simulink model "PID_Roll"  (R2016b)
settings: Solver=ode3  StartTime=0.0  StopTime=20  FixedStep=.02  RelTol=1e-3  EnableMultiTasking=on
InitFcn:
  | close all
  | clear
  | clc
  | Parameter_Modeling
  | ST=0.02;
  | angle_scale=.0109863;  % 1/91.0222
  | time_scale=.01;
undefined symbols (not defined in the file or in its folder): KD_Roll, KI_Roll, KP_Roll
libraries: arduinolib x5
settings Model: SimulationMode=external  ExtModeTrigDuration=2  Creator=Alireza  LastModifiedBy=Ali
settings DataIOCC: LimitDataPoints=on  SaveFormat=Array
settings OptimizationCC: ExpressionDepthLimit=2147483647  MaxStackSize=64
settings DebuggingCC: UnderspecifiedInitializationDetection=Classic  MergeDetectMultiDrivingBlocksExec=none  ParameterTunabilityLossMsg=error  StateNameClashWarn=warning  SFUnexpectedBacktrackingDiag=warning  SFNoUnconditionalDefaultTransitionDiag=warning  SFExecutionAtInitializationDiag=none
settings HardwareCC: ProdBitPerInt=16  ProdBitPerPointer=16  ProdBitPerSizeT=16  ProdBitPerPtrDiffT=16  ProdLargestAtomicFloat=None  ProdWordSize=8  ProdHWDeviceType=Atmel->AVR
settings ModelReferenceCC: PropagateSignalLabelsOutOfModel=off
settings RTWCC: Description=Embedded Coder  SystemTargetFile=ert.tlc  HardwareBoard=Arduino Mega 2560  TLCOptions=-aInlineSetEventsForThisBaseRateFcn=TLC_FALSE -aRateBasedStepFcn=1 -aSuppressMultiTaskScheduler=TLC_FALSE  TemplateMakefile=ert_default_tmf  GenerateReport=on  RTWVerbose=off  Toolchain=Arduino AVR  BuildConfiguration=Faster Runs  IncludeHyperlinkInReport=on  LaunchReport=on  GenerateTraceInfo=on  GenerateTraceReport=on  GenerateTraceReportSl=on  GenerateTraceReportSf=on  GenerateTraceReportEml=on
settings CodeAppCC: ForceParamTrailComments=on  IgnoreCustomStorageClasses=off  OperatorAnnotations=on  SimulinkDataObjDesc=on  SFDataObjDesc=on  MATLABFcnDesc=on  CustomSymbolStrType=$N$R$M  InsertBlockDesc=on  MATLABSourceComments=on  InternalIdentifier=Classic
settings ERTTargetCC: SupportContinuousTime=on  SupportVariableSizeSignals=on
settings ConfigComp: CovMetricSettings=dw  CovHtmlReporting=on  CovSaveCumulativeToWorkspaceVar=on  CovSaveSingleToWorkspaceVar=on  CovExternalEMLEnable=off  CovSFcnEnable=off

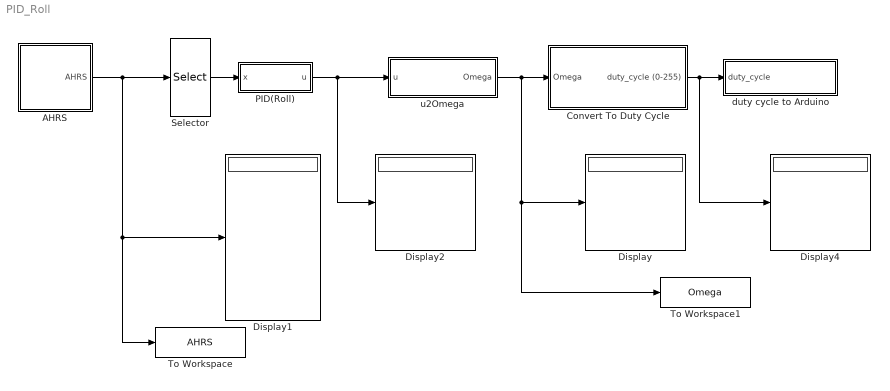
== system PID_Roll ==
  AHRS : Subsystem
      mask Display: image('UM7.jpg'); % Use "Edit Image" on toolstrip to change.
  Convert To Duty Cycle : Subsystem
  Display{,1..2,4} (4 alike) : Display
  PID(Roll) : Subsystem
  Selector : Selector  InputPortWidth=6  IndexOptions=Index vector (dialog)  Indices=[1 4]  OutputSizes=1
  To Workspace : ToWorkspace  VariableName=AHRS  SaveFormat=Timeseries  SampleTime=-1
  To Workspace1 : ToWorkspace  VariableName=Omega  SaveFormat=Timeseries  SampleTime=-1
  duty cycle to Arduino : Subsystem
  u2Omega : Subsystem
  wires:
  u2Omega/1(Omega) -> To Workspace1/1, Display/1, Convert To Duty Cycle/1(Omega)
  PID(Roll)/1(u) -> Display2/1, u2Omega/1(u)
  AHRS/1(AHRS) -> Selector/1, To Workspace/1, Display1/1
  Convert To Duty Cycle/1(duty_cycle (0-255)) -> Display4/1, duty cycle to Arduino/1(duty_cycle)
  Selector/1 -> PID(Roll)/1(x)

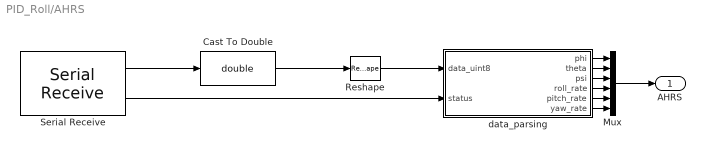
== system PID_Roll/AHRS ==
  Cast To Double : DataTypeConversion  OutDataTypeStr=double
  Mux : Mux  Inputs=6
  Reshape : Reshape
  Serial Receive : arduinolib/Serial Receive  isARMArch=off  portNumber=1  DataType=uint8  Datalength=32  SampleTime=0.02  showOutStatus=on  blockPlatform=arduino
  data_parsing : MATLAB Function  TreatAsAtomicUnit=on
  AHRS : Outport
  wires:
  data_parsing/2(theta) -> Mux/2
  data_parsing/3(psi) -> Mux/3
  data_parsing/4(roll_rate) -> Mux/4
  Reshape/1 -> data_parsing/1(data_uint8)
  data_parsing/5(pitch_rate) -> Mux/5
  Serial Receive/2 -> data_parsing/2(status)
  data_parsing/6(yaw_rate) -> Mux/6
  Cast To Double/1 -> Reshape/1
  Serial Receive/1 -> Cast To Double/1
  data_parsing/1(phi) -> Mux/1
  Mux/1 -> AHRS/1

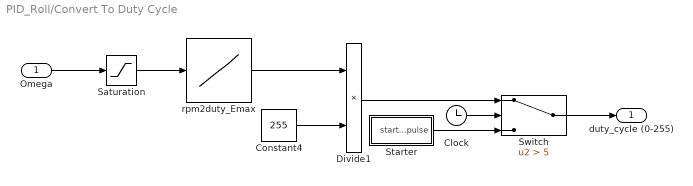
== system PID_Roll/Convert To Duty Cycle ==
  Omega : Inport
  Clock : Clock
  Constant4 : Constant  Value=255
  Divide1 : Product  Inputs=**
  Saturation : Saturate  UpperLimit=6000  LowerLimit=1300
  Starter : Subsystem
  Switch : Switch  Criteria=u2 > Threshold  Threshold=5
  rpm2duty_Emax : Lookup_n-D  NumberOfTableDimensions=1  BreakpointsForDimension1=|  Table=|  RndMeth=Simplest  InputSameDT=on
      BreakpointsForDimension1=|
      | [1201
      | 2305
      | 3096
      | 3930
      | 4118
      | 4555
      | 5122
      | 5552
      | 5957
      | 6291
      | 6360]
      Table=|
      | [0.5
      | 0.55
      | 0.6
      | 0.65
      | 0.7
      | 0.75
      | 0.8
      | 0.85
      | 0.9
      | 0.95
      | 1]
  duty_cycle (0-255) : Outport
  wires:
  Switch/1 -> duty_cycle (0-255)/1
  Clock/1 -> Switch/2
  Divide1/1 -> Switch/1
  rpm2duty_Emax/1 -> Divide1/1
  Starter/1(start_pulse) -> Switch/3
  Omega/1 -> Saturation/1
  Constant4/1 -> Divide1/2
  Saturation/1 -> rpm2duty_Emax/1

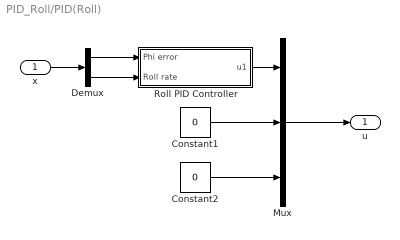
== system PID_Roll/PID(Roll) ==
  x : Inport
  Constant1 : Constant  Value=0
  Constant2 : Constant  Value=0
  Demux : Demux  Outputs=2
  Mux : Mux  Inputs=3
  Roll PID Controller : Subsystem  VariantControl=Choice
  u : Outport
  wires:
  Mux/1 -> u/1
  x/1 -> Demux/1
  Demux/2 -> Roll PID Controller/2(Roll rate)
  Constant2/1 -> Mux/3
  Demux/1 -> Roll PID Controller/1(Phi error)
  Roll PID Controller/1(u1) -> Mux/1
  Constant1/1 -> Mux/2

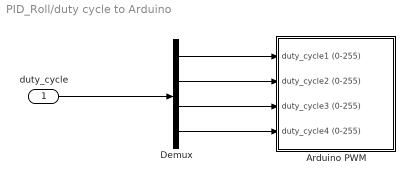
== system PID_Roll/duty cycle to Arduino ==
  duty_cycle : Inport
  Arduino PWM : Subsystem  mask{Motor1=8, Motor2=9, Motor3=10, Motor4=11}
      mask prompts: Motor1 "Motor 1 Pin Number"; Motor2 "Motor 2 Pin Number"; Motor3 "Motor 3 Pin Number"; Motor4 "Motor 4 Pin Number"
  Demux : Demux
  wires:
  duty_cycle/1 -> Demux/1
  Demux/1 -> Arduino PWM/1(duty_cycle1 (0-255))
  Demux/2 -> Arduino PWM/2(duty_cycle2 (0-255))
  Demux/3 -> Arduino PWM/3(duty_cycle3 (0-255))
  Demux/4 -> Arduino PWM/4(duty_cycle4 (0-255))

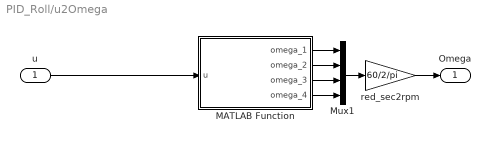
== system PID_Roll/u2Omega ==
  u : Inport
  MATLAB Function : MATLAB Function  TreatAsAtomicUnit=on
  Mux1 : Mux
  red_sec2rpm : Gain  Gain=60/2/pi
  Omega : Outport
  wires:
  Mux1/1 -> red_sec2rpm/1
  MATLAB Function/2(omega_2) -> Mux1/2
  u/1 -> MATLAB Function/1(u)
  MATLAB Function/3(omega_3) -> Mux1/3
  MATLAB Function/1(omega_1) -> Mux1/1
  MATLAB Function/4(omega_4) -> Mux1/4
  red_sec2rpm/1 -> Omega/1

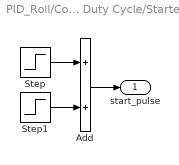
== system PID_Roll/Convert To Duty Cycle/Starter ==
  Add : Sum
  Step : Step  After=140
  Step1 : Step  Time=2  After=-30
  start_pulse : Outport
  wires:
  Add/1 -> start_pulse/1
  Step/1 -> Add/1
  Step1/1 -> Add/2

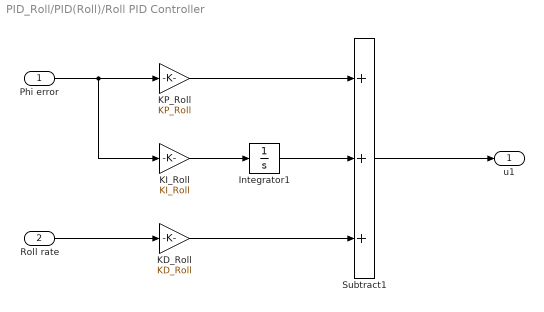
== system PID_Roll/PID(Roll)/Roll PID Controller ==
  Phi error : Inport
  Roll rate : Inport  Port=2
  Integrator1 : Integrator
  KD_Roll : Gain  Gain=KD_Roll
  KI_Roll : Gain  Gain=KI_Roll
  KP_Roll : Gain  Gain=KP_Roll
  Subtract1 : Sum  Inputs=+++
  u1 : Outport
  wires:
  Integrator1/1 -> Subtract1/2
  KI_Roll/1 -> Integrator1/1
  KD_Roll/1 -> Subtract1/3
  Subtract1/1 -> u1/1
  KP_Roll/1 -> Subtract1/1
  Roll rate/1 -> KD_Roll/1
  Phi error/1 -> KI_Roll/1, KP_Roll/1

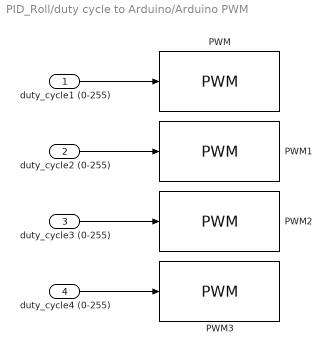
== system PID_Roll/duty cycle to Arduino/Arduino PWM ==
  duty_cycle1 (0-255) : Inport
  duty_cycle2 (0-255) : Inport  Port=2
  duty_cycle3 (0-255) : Inport  Port=3
  duty_cycle4 (0-255) : Inport  Port=4
  PWM : arduinolib/PWM  pinNumber=Motor1  frequencyType=Default  desiredFrequency=490.2  achievableFrequency=490.2
  PWM1 : arduinolib/PWM  pinNumber=Motor2  frequencyType=Default  desiredFrequency=490.2  achievableFrequency=490.2
  PWM2 : arduinolib/PWM  pinNumber=Motor3  frequencyType=Default  desiredFrequency=490.2  achievableFrequency=490.2
  PWM3 : arduinolib/PWM  pinNumber=Motor4  frequencyType=Default  desiredFrequency=490.2  achievableFrequency=490.2
  wires:
  duty_cycle1 (0-255)/1 -> PWM/1
  duty_cycle2 (0-255)/1 -> PWM1/1
  duty_cycle3 (0-255)/1 -> PWM2/1
  duty_cycle4 (0-255)/1 -> PWM3/1

== matlab function PID_Roll/AHRS/data_parsing ==
  data: phi output size=1; data_uint8 input size=32; theta output size=1; psi output size=1; roll_rate output size=1; pitch_rate output size=1; yaw_rate output size=1; status input
function [phi,theta,psi,roll_rate,pitch_rate,yaw_rate] = fcn(data_uint8, status)
persistent stepp check_sum...
    phi_p theta_p psi_p roll_rate_p pitch_rate_p yaw_rate_p...
    phi_last theta_last psi_last roll_rate_last pitch_rate_last yaw_rate_last;
%% Initialize
if isempty(stepp)
    stepp=0;
    check_sum=0;
    phi_p=0;
    theta_p=0;
    psi_p=0;
    roll_rate_p=0;
    pitch_rate_p=0;
    yaw_rate_p=0;
    phi_last=0;
    theta_last=0;
    psi_last=0;
    roll_rate_last=0;
    pitch_rate_last=0;
    yaw_rate_last=0;
end
angle_scale=.0109863;  % 1/91.0222
rate_scale=1/16;
%% Check Each Byte
if status
    for i = 1:length(data_uint8)
        if (data_uint8(i)==115 && stepp==0)
            stepp=1;
            check_sum=data_uint8(i);
        elseif(stepp==1 && data_uint8(i)==110)
            stepp=stepp+1;
            check_sum=check_sum+data_uint8(i);
        elseif(stepp==2 && data_uint8(i)==112)
            stepp=stepp+1;
            check_sum=check_sum+data_uint8(i);
        elseif(stepp==3 && data_uint8(i)==212)
            stepp=stepp+1;
            check_sum=check_sum+data_uint8(i);
        elseif(stepp==4 && data_uint8(i)==112)
            stepp=stepp+1;
            check_sum=check_sum+data_uint8(i);
        elseif(stepp==5)
            phi_p=data_uint8(i)*256;
            stepp=stepp+1;
            check_sum=check_sum+data_uint8(i);
        elseif(stepp==6)
            phi_p=phi_p+data_uint8(i);
            stepp=stepp+1;
            check_sum=check_sum+data_uint8(i);
        elseif(stepp==7)
            theta_p=data_uint8(i)*256;
            stepp=stepp+1;
            check_sum=check_sum+data_uint8(i);
        elseif(stepp==8)
            theta_p=theta_p+data_uint8(i);
            stepp=stepp+1;
            check_sum=check_sum+data_uint8(i);
        elseif(stepp==9)
            psi_p=data_uint8(i)*256;
            stepp=stepp+1;
            check_sum=check_sum+data_uint8(i);
        elseif(stepp==10)
            psi_p=psi_p+data_uint8(i);
            stepp=stepp+1;
            check_sum=check_sum+data_uint8(i);
        elseif(stepp==11 || stepp==12)
            if(data_uint8(i)==0)
                stepp=stepp+1;
            else
                stepp=0;
            end
        elseif(stepp==13)
            roll_rate_p=data_uint8(i)*256;
            stepp=stepp+1;
            check_sum=check_sum+data_uint8(i);
        elseif(stepp==14)
            roll_rate_p=roll_rate_p+data_uint8(i);
            stepp=stepp+1;
            check_sum=check_sum+data_uint8(i);
        elseif(stepp==15)
            pitch_rate_p=data_uint8(i)*256;
            stepp=stepp+1;
            check_sum=check_sum+data_uint8(i);
        elseif(stepp==16)
            pitch_rate_p=pitch_rate_p+data_uint8(i);
            stepp=stepp+1;
            check_sum=check_sum+data_uint8(i);
        elseif(stepp==17)
            yaw_rate_p=data_uint8(i)*256;
            stepp=stepp+1;
            check_sum=check_sum+data_uint8(i);
        elseif(stepp==18)
            yaw_rate_p=yaw_rate_p+data_uint8(i);
            stepp=stepp+1;
            check_sum=check_sum+data_uint8(i);
        elseif(stepp==19 || stepp==20)
            if(data_uint8(i)==0)
                stepp=stepp+1;
            else
                stepp=0;
            end
        elseif(stepp==21 || stepp==22 || stepp==23 || stepp==24)
            stepp=stepp+1;
            check_sum=check_sum+data_uint8(i);
        elseif(stepp==25)
            if (floor(check_sum/256)==data_uint8(i))
                stepp=stepp+1;
            else
                stepp=0;
            end
        elseif(stepp==26)
            if(mod(check_sum,256)==data_uint8(i))
                phi_last=double(typecast(uint16(phi_p), 'int16'))*angle_scale;
                if mod(phi_last,360)>180
                    phi_last=mod(phi_last,360)-360;
                else
                    phi_last=mod(phi_last,360);
                end
                theta_last=double(typecast(uint16(theta_p), 'int16'))*angle_scale;
                if mod(theta_last,360)>180
                    theta_last=mod(theta_last,360)-360;
                else
                    theta_last=mod(theta_last,360);
                end
                psi_last=double(typecast(uint16(psi_p), 'int16'))*angle_scale;
                if mod(psi_last,360)>180
                    psi_last=mod(psi_last,360)-360;
                else
                    psi_last=mod(psi_last,360);
                end
                roll_rate_last=double(typecast(uint16(roll_rate_p), 'int16'))*rate_scale;
                if mod(roll_rate_last,360)>180
                    roll_rate_last=mod(roll_rate_last,360)-360;
                else
                    roll_rate_last=mod(roll_rate_last,360);
                end
                pitch_rate_last=double(typecast(uint16(pitch_rate_p), 'int16'))*rate_scale;
                if mod(pitch_rate_last,360)>180
                    pitch_rate_last=mod(pitch_rate_last,360)-360;
                else
                    pitch_rate_last=mod(pitch_rate_last,360);
                end
                yaw_rate_last=double(typecast(uint16(yaw_rate_p), 'int16'))*rate_scale;
                if mod(yaw_rate_last,360)>180
                    yaw_rate_last=mod(yaw_rate_last,360)-360;
                else
                    yaw_rate_last=mod(yaw_rate_last,360);
                end
            end
            stepp=0;
        end
    end
end

%% Assign Last True Data to Output
phi=phi_last;
theta=theta_last;
psi=psi_last;
roll_rate=roll_rate_last;
pitch_rate=pitch_rate_last;
yaw_rate=yaw_rate_last;

== matlab function PID_Roll/u2Omega/MATLAB Function ==
  data: u input; omega_1 output; omega_2 output; omega_3 output; omega_4 output
function [omega_1, omega_2, omega_3, omega_4] = fcn(u)
u1 = u(1);
u2 = u(2);
u3 = u(3);
% control effort
u4 = ones(1, length(u1)) * 4 * rpm2rad_sec(2000)^2;
% calculate omega
if (u4 + u3 + 2 * u2) < 0
    omega_1 = 0;
else
    omega_1 = sqrt((u4 + u3 + 2 * u2) / 4);
end
if (u4 + u3 - 2 * u2) < 0
    omega_3 = 0;
else
    omega_3 = sqrt((u4 + u3 - 2 * u2) / 4);
end
if (u4 - u3 + 2 * u1) < 0
    omega_2 = 0;
else
    omega_2 = sqrt((u4 - u3 + 2 * u1) / 4);
end
if (u4 - u3 - 2 * u1) < 0
    omega_4 = 0;
else
    omega_4 = sqrt((u4 - u3 - 2 * u1) / 4);
end
end
%% functions
% rpm to rad/sec
function rad = rpm2rad_sec(rpm)
rad = rpm / 60 * 2 * pi;
end
